simulink model "product_matrix_multiple_test_2"  (R2017b)
settings: Solver=FixedStepAuto  StartTime=0.0  StopTime=10.0  FixedStep=0.1  RelTol=1e-3  EnableMultiTasking=on
model workspace (MAT data in the model file):
  lustrec_slx_eps = 100
settings Model: Creator=arnaud  LastModifiedBy=hbourbou
settings DataIOCC: LimitDataPoints=on  SaveFormat=Structure  SignalLoggingSaveFormat=ModelDataLogs
settings OptimizationCC: ExpressionDepthLimit=2147483647  LifeSpan=inf
settings DebuggingCC: UnderspecifiedInitializationDetection=Classic  MergeDetectMultiDrivingBlocksExec=none  SolverPrmCheckMsg=warning  FcnCallInpInsideContextMsg=warning  StateNameClashWarn=warning  SFUnexpectedBacktrackingDiag=warning  SFNoUnconditionalDefaultTransitionDiag=warning  SFExecutionAtInitializationDiag=none
settings HardwareCC: ProdBitPerPointer=32  ProdBitPerSizeT=32  ProdBitPerPtrDiffT=32  ProdLargestAtomicFloat=None  ProdIntDivRoundTo=Undefined  ProdEndianess=Unspecified  ProdWordSize=32  ProdHWDeviceType=32-bit Generic
settings ModelReferenceCC: PropagateSignalLabelsOutOfModel=off
settings CodeAppCC: StateflowObjectComments=on
settings GRTTargetCC: TargetLangStandard=C89/C90 (ANSI)  GeneratePreprocessorConditionals=Disable all  CombineOutputUpdateFcns=off  GRTInterface=on
settings ConfigComp: CovMetricSettings=dw  CovHtmlReporting=on  CovSaveCumulativeToWorkspaceVar=on  CovSaveSingleToWorkspaceVar=on  CovExternalEMLEnable=off  CovSFcnEnable=off

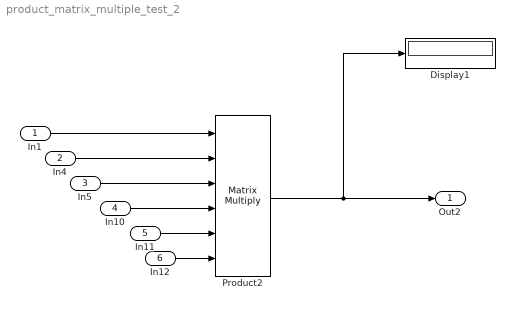
== system product_matrix_multiple_test_2 ==
  In1 : Inport  OutMin=-1.  OutMax=1.  OutDataTypeStr=double  PortDimensions=[2 4]
  In4 : Inport  Port=2  OutMin=-2.  OutMax=2.  OutDataTypeStr=double  PortDimensions=[4 2]
  In5 : Inport  Port=3  OutMin=-1.  OutMax=1.  OutDataTypeStr=double  PortDimensions=[2 3]
  In10 : Inport  Port=4  OutMin=-2.  OutMax=1.  OutDataTypeStr=double  PortDimensions=[3 3]
  In11 : Inport  Port=5  OutMin=-1.  OutMax=.5  OutDataTypeStr=double  PortDimensions=[3 2]
  In12 : Inport  Port=6  OutMin=-3.  OutMax=-1.  OutDataTypeStr=double  PortDimensions=[2 1]
  Display1 : Display
  Product2 : Product  Inputs=6  Multiplication=Matrix(*)  RndMeth=Zero
  Out2 : Outport
  wires:
  In1/1 -> Product2/1
  Product2/1 -> Display1/1, Out2/1
  In4/1 -> Product2/2
  In5/1 -> Product2/3
  In10/1 -> Product2/4
  In11/1 -> Product2/5
  In12/1 -> Product2/6
